simulink library "MX_Library"  (Simulink 7.7)
settings: Solver=ode45  StartTime=0.0  StopTime=10.0  RelTol=1e-3
values from neighbouring files (symbols this model uses):
  ACTIVE = Bobcat.Parameter; CreateDefine( ACTIVE                         ,1                          ,'Define' ,'defines.h' )    [defines.m]
  CD_PRECISION_REF_NOMINAL_VALUE = Bobcat.Parameter; CreateAliasCD( CD_PRECISION_REF_NOMINAL_VALUE                       ,uint16(511)                ,'ConstantDataPointer' ,'CONSTANT_DATA' ,'PRECISION_REF_NOMINAL_VALUE')    [cdata.m]
  ENGINE_CRANKING = Bobcat.Parameter; CreateDefine( ENGINE_CRANKING                ,2                          ,'Define' ,'defines.h' )    [defines.m]
  ERROR_OFF = Bobcat.Parameter; CreateDefine( ERROR_OFF                      ,3                          ,'Define' ,'defines.h' )    [defines.m]
  ERROR_ON = Bobcat.Parameter; CreateDefine( ERROR_ON                       ,2                          ,'Define' ,'defines.h' )    [defines.m]
  FAILURE = Bobcat.Parameter; CreateDefine( FAILURE                        ,28                         ,'Define' ,'defines.h' )    [defines.m]
  FULL_ON = Bobcat.Parameter; CreateDefine( FULL_ON                        ,fi(0,0,16,16,'hex','ffff') ,'Define' ,'defines.h' )    [defines.m]
  INACTIVE = Bobcat.Parameter; CreateDefine( INACTIVE                       ,0                          ,'Define' ,'defines.h' )    [defines.m]
  NON_FUNCTIONAL = Bobcat.Parameter; CreateDefine( NON_FUNCTIONAL                 ,255                        ,'Define' ,'defines.h' )    [defines.m]
  NORMAL = Bobcat.Parameter; CreateDefine( NORMAL                         ,8                          ,'Define' ,'defines.h' )    [defines.m]
  OORL = Bobcat.Parameter; CreateDefine( OORL                           ,22                         ,'Define' ,'defines.h' )    [defines.m]
  OPEN_CIRCUIT = Bobcat.Parameter; CreateDefine( OPEN_CIRCUIT                   ,7                          ,'Define' ,'defines.h' )    [defines.m]
  OPEN_STG = Bobcat.Parameter; CreateDefine( OPEN_STG                       ,31                         ,'Define' ,'defines.h' )    [defines.m]
  OVERCURRENT = Bobcat.Parameter; CreateDefine( OVERCURRENT                    ,32                         ,'Define' ,'defines.h' )    [defines.m]
  RESET = Bobcat.Parameter; CreateDefine( RESET                          ,2                          ,'Define' ,'defines.h' )    [defines.m]
  SHORT_TO_BATTERY = Bobcat.Parameter; CreateDefine( SHORT_TO_BATTERY               ,5                          ,'Define' ,'defines.h' )    [defines.m]
  SHORT_TO_GROUND = Bobcat.Parameter; CreateDefine( SHORT_TO_GROUND                ,6                          ,'Define' ,'defines.h' )    [defines.m]
  srate = 0.010    (= 0.01)    [LoadWorkspace.m]
  UNLIMITED = Bobcat.Parameter; CreateDefine( UNLIMITED                      ,65535                      ,'Define' ,'defines.h' )    [defines.m]
undefined symbols (not defined in the file or in its folder): BIDIRECTIONAL_CTRL, CD__AFBK_GAIN, CD__DEBOUNCE_OPEN_CIRCUIT, CD__DEBOUNCE_OVERCURRENT, CD__DEBOUNCE_SHORT_TO_BATTERY, CD__DEBOUNCE_SHORT_TO_GROUND, CD__ENABLE_AFBK_GAIN, CD__ENABLE_DEBOUNCE_OPEN_CIRCUIT, CD__ENABLE_DEBOUNCE_OVERCURRENT, CD__ENABLE_DEBOUNCE_SHORT_TO_BATTERY, CD__ENABLE_DEBOUNCE_SHORT_TO_GROUND, CD__ENABLE_FEEDBACK_FUNCTION, CD__ENABLE_IFBK_GAIN, CD__ENABLE_MAX_VOLTS, CD__ENABLE_NON_ZERO_CURRENT, CD__ENABLE_NON_ZERO_DUTY, CD__ENABLE_OVERCURRENT, CD__FUNCTION, CD__IFBK_GAIN, CD__KI, CD__KP, CD__MAX_VOLTS, CD__NON_ZERO_CURRENT, CD__NON_ZERO_DUTY, CD__OVERCURRENT, DEBOUNCE_ERROR_OFF, DEBOUNCE_ERROR_ON, DiscIntNeverNeededParam, FN_, IFBK_MAX, KI, KP, MAX_VOLTS, NZ_DUTY, NZ_IFBK, OC_DB_CNT, OPEN_DB_CNT, OSTG_DB_CNT, STB_DB_CNT, STG_DB_CNT
libraries: simulink x12, MX_Library x11
(part 1 of 2)
settings Model: Creator=alliebel  LastModifiedBy=aliebel

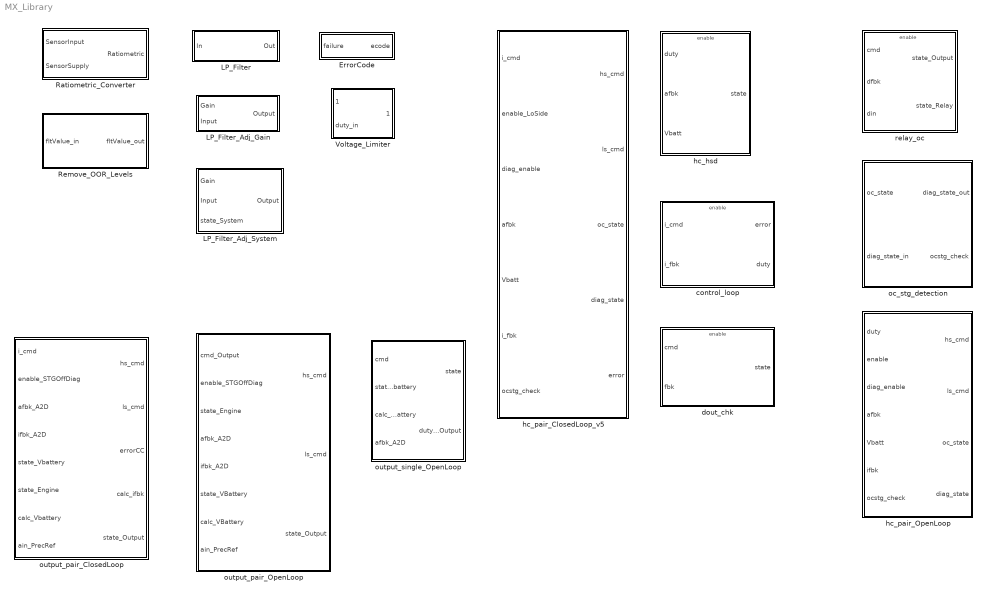
== system MX_Library ==
  ErrorCode : Subsystem  TreatAsAtomicUnit=on  RTWFileName=mod_Library  mask{FUNCTION=FN_}
      settings: AttributesFormatString=FUNCTION=%<FUNCTION>  RTWFcnNameOpts=Use subsystem name  RTWFileNameOpts=User specified
  LP_Filter : Subsystem  TreatAsAtomicUnit=on  RTWFcnName=LP_Filter  RTWFileName=mod_Library  mask{GAIN=3}
      mask prompts: GAIN "Gain for filter"
      settings: RTWFcnNameOpts=Use subsystem name  RTWFileNameOpts=User specified
  LP_Filter_Adj_Gain : Subsystem  TreatAsAtomicUnit=on  RTWFileName=mod_Library
      settings: RTWFcnNameOpts=Use subsystem name  RTWFileNameOpts=User specified
  LP_Filter_Adj_System : Subsystem  TreatAsAtomicUnit=on  RTWFileName=mod_Library
      settings: RTWFcnNameOpts=Use subsystem name  RTWFileNameOpts=User specified
  Ratiometric_Converter : Subsystem  TreatAsAtomicUnit=on  RTWFileName=mod_Library  mask{multiplier=1000}
      mask prompts: multiplier "Ratiometric Multiplier"
      settings: RTWFcnNameOpts=Use subsystem name  RTWFileNameOpts=User specified
  Remove_OOR_Levels : Subsystem  TreatAsAtomicUnit=on  RTWFileName=mod_Library  mask{OORL_LEVEL=50, OORH_LEVEL=950}
      settings: RTWFcnNameOpts=Use subsystem name  RTWFileNameOpts=User specified
  Voltage_Limiter : Subsystem  TreatAsAtomicUnit=on  RTWFileName=mod_Library
      settings: RTWFileNameOpts=User specified
  control_loop : Subsystem  TreatAsAtomicUnit=on  RTWFileName=mod_Library  mask{KP=KP, KI=KI}
      mask prompts: KP "Proportional Gain (Kp) -storage: fi(1,16,15)"; KI "Integral Gain (Ki) -storage: fi(1,16,15)"
      settings: RTWFcnNameOpts=Use subsystem name  RTWFileNameOpts=User specified
  dout_chk : Subsystem  TreatAsAtomicUnit=on  mask(Low Current, Low Side Driver -Monitor){ERR_ON_DB_CNT=DEBOUNCE_ERROR_ON, ERR_OFF_DB_CNT=DEBOUNCE_ERROR_OFF}
      mask prompts: ERR_ON_DB_CNT "Error On debounce count (10mS/count)"; ERR_OFF_DB_CNT "Error Off debounce count (10mS/count)"
      mask help:
      | Inputs:
      |   cmd: current output command (0-off, 1-on)
      |       storage: boolean
      |
      |   fbk: current output feedback (0-off, 1-on)
      |       storage: boolean
      |
      | Outputs:
      |   state:   8-bit value representing driver state
      |             (8) -> OK
      |             (2) -> error on   // cmd==off, fbk==on
      |             (3) -> error off  // cmd==on,  fbk==off
      mask Help: This block monitors the state of a digital output.
  hc_hsd : Subsystem  TreatAsAtomicUnit=on  RTWFileName=mod_Library  mask(High Current, High Side Driver -Monitor){STB_DB_CNT=STB_DB_CNT, STG_DB_CNT=STG_DB_CNT, OPEN_DB_CNT=OPEN_DB_CNT}
      mask prompts: STB_DB_CNT "Short to Battery (STB) debounce count"; STG_DB_CNT "Short to Ground (STG) debounce count"; OPEN_DB_CNT "Open circuit debounce count"
      mask help:
      | Inputs:
      |     duty: current output command (pwm %,  0-off, 1-on)
      |            storage:  ufix(16) - 100 / (2^16-1) percent per bit.
      |
      |     afbk:  high side analog feedback (volts)
      |            storage:  ufix(16) - 1 / (2^8)  volts per bit.
      |
      |     Vbatt: battery potential (volts)
      |            storage:  ufix(16) - 1 / (2^8)  volts per bit.
      |
      | Outputs:
      |     state:  8-bit value representing detected fault condition.
      |                (8) -> OK, output operating properly.
      |                (5) -> STB, short to battery
      |                (6) -> STG, short to ground
      |                (7) -> OPEN, open circuit
      settings: RTWFcnNameOpts=Use subsystem name  RTWFileNameOpts=User specified
      mask Help:
      | This block monitors the feedbacks associated with a "hc_hsd" (hig-current high-side-driver) and reports any faults associated with the output.
      | 
      | Parameter storage.
      | 
      | STB_DB_CNT : ufix(16) - 0.01 seconds per bit.
  hc_pair_ClosedLoop_v5 : Subsystem  TreatAsAtomicUnit=on  RTWFileName=mod_Library  mask{IFBK_MAX=IFBK_MAX, NZ_IFBK=NZ_IFBK, NZ_DUTY=NZ_DUTY, STB_DB_CNT=STB_DB_CNT, OPEN_DB_CNT=OPEN_DB_CNT, OSTG_DB_CNT=OSTG_DB_CNT, STG_DB_CNT=STG_DB_CNT, OC_DB_CNT=OC_DB_CNT, KP=KP, KI=KI, BIDIRECTIONAL_CTRL=BIDIRECTIONAL_CTRL}
      mask prompts: IFBK_MAX "Over Current Limit (Amps)  -storage uint(16), 1/2^12 amps per bit."; NZ_IFBK "Non-Zero Current (Amps) -storage uint(16), 1/2^12 amps per bit"; NZ_DUTY "Non-Zero Duty Cycle (%) -storage uint(16) 100/2^16 % per bit"; STB_DB_CNT "Short To Battery (STB) debounce count -storage uint(16)"; OPEN_DB_CNT "Open debounce count (10mS/count) -storage uint(16)"; OSTG_DB_CNT "Open or Short to Ground (OSTG) debounce count  -storage uint(16)"; STG_DB_CNT "Short To Ground (STG) debounce count -storage uint(16)"; OC_DB_CNT "Over Current (OC) debounce count -storage uint(16)"; KP "Kp  -storage: fi(1,16,15)"; KI "Ki    -storage: fi(1,16,15)C"; BIDIRECTIONAL_CTRL "Bi-directional Current Control"
      mask help:
      | This block implements an open loop High/Low output pair.
      |
      | Inputs:
      |   i_cmd:   command (Amps)...   storage:  ufix(16) - 1/ (2^12) Amps per bit.
      |   enable:    state of output (0-off, 1-on)...   storage: boolean.
      |   diag_enable:    state of diagnostics (0-off, 1-on)...   storage: boolean
      |   afbk:    high side analog feedback (volts)... storage: uint(16) 1/2^8 volts per bit
      |   Vbatt:   battery potential (volts)... storage: uint(16) 1/2^8 volts per bit
      |   ifbk:    low side current feedback (amps)... storage: uint(16) 1/2^12 amps per bit
      |
      | Outputs:
      |     hs_cmd: (pwm%, 0-off, 1-on)...   storage:  ufix(16) - 100/ (2^16-1) percent per bit.
      |     ls_cmd:  (boolean)... storage: boolean
      |     oc_state: state of the over-current detection mechanism.
      |                 (8)  -> Ok
      |                 (32) -> error, too much current sensed flowing through this output
      |                                      output is turned off...
      |
      |   diag_state:  state of the general fault state monitoring.
      |                 (8)  -> Ok
      |                 (5)  -> STB, Short to battery
      |                 (6)  -> STG, Short to ground
      |                 (7)  -> Open, open circuit
      |                 (31) -> OSTG, open or short to ground
      settings: RTWFcnNameOpts=Use subsystem name  RTWFileNameOpts=User specified
  hc_pair_OpenLoop : Subsystem  TreatAsAtomicUnit=on  RTWFileName=mod_Library  mask(hc_pair output){IFBK_MAX=IFBK_MAX, NZ_IFBK=NZ_IFBK, NZ_DUTY=NZ_DUTY, STB_DB_CNT=STB_DB_CNT, OPEN_DB_CNT=OPEN_DB_CNT, OSTG_DB_CNT=OSTG_DB_CNT, STG_DB_CNT=STG_DB_CNT, OC_DB_CNT=OC_DB_CNT}
      mask prompts: IFBK_MAX "Over-Current shutdown limit (Amps)  -storage: uint(16) 1/2^12 amps/bit"; NZ_IFBK "Non-Zero current feedback (Amps) -storage: uint(16) 1/2^12 amps/bit"; NZ_DUTY "Non-Zero duty cycle (% duty) -storage uint(16) 100/2^16 % per bit."; STB_DB_CNT "Short to Battey (STB) debounce count -storage uint(16)"; OPEN_DB_CNT "Open debounce count -storage uint(16)"; OSTG_DB_CNT "Open or short to Ground (OSTG) debounce count -storage uint(16)"; STG_DB_CNT "Short to Ground (STG) debounce count -storage uint(16)"; OC_DB_CNT "Overcurrent debounce count -storage uint(16)"
      mask help:
      | This block implements an open loop High/Low output pair.
      |
      | Inputs:
      |   duty:    pwm%, 0-off, 1-on)...   storage:  ufix(16) - 100/ (2^16-1) percent per bit.
      |   enable:    state of output (0-off, 1-on)...   storage: boolean.
      |   diag_enable:    state of diagnostics (0-off, 1-on)...   storage: boolean
      |   afbk:    high side analog feedback (volts)... storage: uint(16) 1/2^8 volts per bit
      |   Vbatt:   battery potential (volts)... storage: uint(16) 1/2^8 volts per bit
      |   ifbk:    low side current feedback (amps)... storage: uint(16) 1/2^12 amps per bit
      |
      | Outputs:
      |     hs_cmd: (pwm%, 0-off, 1-on)...   storage:  ufix(16) - 100/ (2^16-1) percent per bit.
      |     ls_cmd:  (boolean)... storage: boolean
      |     oc_state: state of the over-current detection mechanism.
      |                 (8)  -> Ok
      |                 (32) -> error, too much current sensed flowing through this output
      |                                      output is turned off...
      |
      |   diag_state:  state of the general fault state monitoring.
      |                 (8)  -> Ok
      |                 (5)  -> STB, Short to battery
      |                 (6)  -> STG, Short to ground
      |                 (7)  -> Open, open circuit
      |                 (31) -> OSTG, open or short to ground
      settings: RTWFcnNameOpts=Use subsystem name  RTWFileNameOpts=User specified
  oc_stg_detection : Subsystem  TreatAsAtomicUnit=on  RTWFileName=mod_Library  mask{CD_DEBOUNCE_OPEN_CIRCUIT=OPEN_DB_CNT, CD_DEBOUNCE_SHORT_TO_GROUND=STG_DB_CNT}
      mask prompts: CD_DEBOUNCE_OPEN_CIRCUIT "Debounce Open Circuit"; CD_DEBOUNCE_SHORT_TO_GROUND "Debounce Short to Ground"
      settings: RTWFcnNameOpts=Use subsystem name  RTWFileNameOpts=User specified
  output_pair_ClosedLoop : Subsystem  TreatAsAtomicUnit=on  RTWFileName=mod_Library  mask{AFBK_GAIN=CD__AFBK_GAIN, IFBK_GAIN=CD__IFBK_GAIN, OPEN_DB_CNT=CD__DEBOUNCE_OPEN_CIRCUIT, STG_DB_CNT=CD__DEBOUNCE_SHORT_TO_GROUND, OSTG_DB_CNT=CD__DEBOUNCE_SHORT_TO_GROUND, STB_DB_CNT=CD__DEBOUNCE_SHORT_TO_BATTERY, OC_DB_CNT=CD__DEBOUNCE_OVERCURRENT, IFBK_MAX=CD__OVERCURRENT, NZ_IFBK=CD__NON_ZERO_CURRENT, NZ_DUTY=CD__NON_ZERO_DUTY, KP=CD__KP, KI=CD__KI, BIDIRECTIONAL_CTRL=NON_FUNCTIONAL}
      mask prompts: AFBK_GAIN "Analog Feedback Gain -storage: fi(0,16,8)"; IFBK_GAIN "Current Feedback Gain  -storage: fi(0,16,16)"; OPEN_DB_CNT "Debounce Open Circuit  -storage: uint(16)"; STG_DB_CNT "Debounce STG  -storage uint(16)"; OSTG_DB_CNT "Debounce Open or STG -storage uint(16)"; STB_DB_CNT "Debounce STB -storage uint(16)"; OC_DB_CNT "Debounce Overcurrent -storage uint(16)"; IFBK_MAX "Overcurrent Shutdown limit -storage: fi(0,16,12)"; NZ_IFBK "Non-zero Current Feedback -storage: fi(0,16,12)"; NZ_DUTY "Non-zero Duty Cycle -storage: fi(0,16,16)"; KP "Proportional Gain (Kp) - storage: fi(1,16,15)"; KI "Integral Gain (Ki) - storage: fi(1,16,15)"; BIDIRECTIONAL_CTRL "Bi-Directional Current Control"
      settings: RTWFcnNameOpts=Use subsystem name  RTWFileNameOpts=User specified
  output_pair_OpenLoop : Subsystem  TreatAsAtomicUnit=on  RTWFileName=mod_Library  mask{FEEDBACK_ENABLE=CD__ENABLE_FEEDBACK_FUNCTION, AFBK_GAIN=CD__ENABLE_AFBK_GAIN, IFBK_GAIN=CD__ENABLE_IFBK_GAIN, OPEN_DB_CNT=CD__ENABLE_DEBOUNCE_OPEN_CIRCUIT, STG_DB_CNT=CD__ENABLE_DEBOUNCE_SHORT_TO_GROUND, STB_DB_CNT=CD__ENABLE_DEBOUNCE_SHORT_TO_BATTERY, OC_DB_CNT=CD__ENABLE_DEBOUNCE_OVERCURRENT, OSTG_DB_CNT=CD__ENABLE_DEBOUNCE_SHORT_TO_GROUND, IFBK_MAX=CD__ENABLE_OVERCURRENT, NZ_IFBK=CD__ENABLE_NON_ZERO_CURRENT, NZ_DUTY=CD__ENABLE_NON_ZERO_DUTY, MAX_VOLTS=CD__ENABLE_MAX_VOLTS}
      mask prompts: FEEDBACK_ENABLE "Feedback Enable:"; AFBK_GAIN "Analog Feedback Gain -storage: fi(0,16,8)"; IFBK_GAIN "Current Feedback Gain  -storage: fi(0,16,16)"; OPEN_DB_CNT "Debounce Open Circuit  -storage: uint(16)"; STG_DB_CNT "Debounce STG  -storage uint(16)"; STB_DB_CNT "Debounce STB -storage uint(16)"; OC_DB_CNT "Debounce Overcurrent -storage uint(16)"; OSTG_DB_CNT "Debounce Open or STG -storage uint(16)"; IFBK_MAX "Overcurrent Shutdown limit -storage: fi(0,16,12)"; NZ_IFBK "Non-zero Current Feedback -storage: fi(0,16,12)"; NZ_DUTY "Non-zero Duty Cycle -storage: fi(0,16,16)"; MAX_VOLTS "Maximum Voltage Limit"
      settings: RTWFcnNameOpts=Use subsystem name  RTWFileNameOpts=User specified
  output_single_OpenLoop : Subsystem  TreatAsAtomicUnit=on  RTWFileName=mod_Library  mask{FUNCTION=CD__FUNCTION, AFBK_GAIN=CD__AFBK_GAIN, OPEN_DB_CNT=CD__DEBOUNCE_OPEN_CIRCUIT, STB_DB_CNT=CD__DEBOUNCE_SHORT_TO_BATTERY, STG_DB_CNT=CD__DEBOUNCE_SHORT_TO_GROUND, MAX_VOLTS=CD__MAX_VOLTS}
      mask prompts: FUNCTION "Functional:"; AFBK_GAIN "Analog Feedback Gain: -storage: fi(0,16,8)"; OPEN_DB_CNT "Debounce Open Circuit: -storage: uint(16)"; STB_DB_CNT "Debounce STB: -storage: uint(16)"; STG_DB_CNT "Debounce STG: -storage: uint(16)"; MAX_VOLTS "Maximum Voltage Limit"
      settings: RTWFcnNameOpts=Use subsystem name  RTWFileNameOpts=User specified
  relay_oc : Subsystem  TreatAsAtomicUnit=on  RTWFileName=mod_Library  mask(relay moniitor){ERROR_ON_DB_CNT=40, ERROR_OFF_DB_CNT=40, NORMAL_DB_CNT=40}
      mask prompts: ERROR_ON_DB_CNT "dfbk Error on debounce count"; ERROR_OFF_DB_CNT "dfbk Error off debounce count"; NORMAL_DB_CNT "dfbk normal debounce count"
      mask help:
      | Often "lc_lsd" outputs are used to drive relays.  If this is the case the output of the relay is fed back to a digital input (din) to monitor the relay function.  This block adds the relay output monitor to the "lc_lsd" monitor to create a "relay" monitor.
      |
      | Inputs:
      |   cmd: output command (0-off, 1-on)
      |       storage: boolean
      |
      |   dfbk: output feedback (0-off, 1-on)
      |       storage: boolean
      |
      |   din: relay output feedback (0-off, 1-on)
      |       storage: boolean
      |
      | Outputs:
      |   state:   8-bit value representing driver state
      |             (8) -> OK
      |             (2) -> error on   // cmd==off, dfbk==on
      |             (3) -> error off  // cmd==on,  dfbk==off
      |
      |   din_state:   8-bit value representing driver state
      |             (8) -> OK
      |             (2) -> error on   // cmd==off, din==on
      |             (3) -> error off  // cmd==on,  din==off
      settings: RTWFcnNameOpts=Use subsystem name  RTWFileNameOpts=User specified

== system MX_Library/ErrorCode ==
  failure : Inport  OutDataTypeStr=uint8
  Constant : Constant  Value=256  OutDataTypeStr=uint16
  Constant1 : Constant  Value=FUNCTION  OutDataTypeStr=uint16
  Product : Product  OutDataTypeStr=uint16  RndMeth=Zero
  Sum : Sum  OutDataTypeStr=uint16
  ecode : Outport  OutDataTypeStr=uint16
  wires:
  Constant/1 -> Product/2
  Constant1/1 -> Product/1
  Product/1 -> Sum/2
  failure/1 -> Sum/1
  Sum/1 -> ecode/1

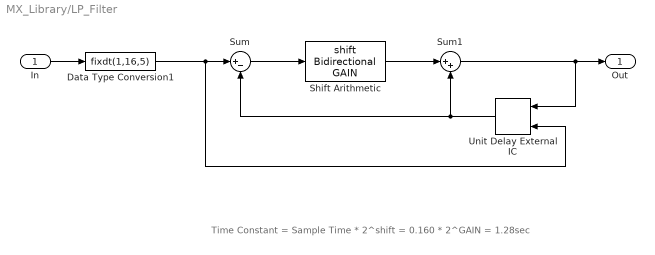
== system MX_Library/LP_Filter ==
  note: Time Constant = Sample Time * 2^shift
      | = 0.160 * 2^GAIN = 1.28sec
  In : Inport
  Data Type Conversion1 : DataTypeConversion  OutMin=0  OutMax=1023  OutDataTypeStr=fixdt(1,16,5)
  Shift Arithmetic : ArithShift  BitShiftNumber=GAIN
  Sum : Sum  Inputs=|+-  OutDataTypeStr=fixdt(1,16,5)  SaturateOnIntegerOverflow=on
  Sum1 : Sum  Inputs=|++  OutDataTypeStr=fixdt(1,16,5)  SaturateOnIntegerOverflow=on
  Unit Delay External IC : simulink/Additional Math & Discrete/Additional Discrete/Unit Delay External IC  SystemSampleTime=-1  tsamp=-1
  Out : Outport
  wires:
  Sum/1 -> Shift Arithmetic/1
  Sum1/1 -> Unit Delay External IC/1, Out/1
  Shift Arithmetic/1 -> Sum1/1
  Unit Delay External IC/1 -> Sum1/2, Sum/2
  In/1 -> Data Type Conversion1/1
  Data Type Conversion1/1 -> Sum/1, Unit Delay External IC/2

== system MX_Library/LP_Filter_Adj_Gain ==
  Gain : Inport
  Input : Inport  Port=2
  LP_Filter_Adj_Gain : Stateflow chart  RTWFileName=mod_Library
  Output : Outport
  wires:
  LP_Filter_Adj_Gain/1(Output) -> Output/1
  Input/1 -> LP_Filter_Adj_Gain/2(Input)
  Gain/1 -> LP_Filter_Adj_Gain/1(Gain)

== system MX_Library/LP_Filter_Adj_System ==
  Gain : Inport
  Input : Inport  Port=2
  state_System : Inport  Port=3
  LP_Fitler_Adj_Gain : Stateflow chart  TreatAsAtomicUnit=on
  Output : Outport
  wires:
  state_System/1 -> LP_Fitler_Adj_Gain/3(state_System)
  Gain/1 -> LP_Fitler_Adj_Gain/1(Gain)
  Input/1 -> LP_Fitler_Adj_Gain/2(Input)
  LP_Fitler_Adj_Gain/1(Output) -> Output/1

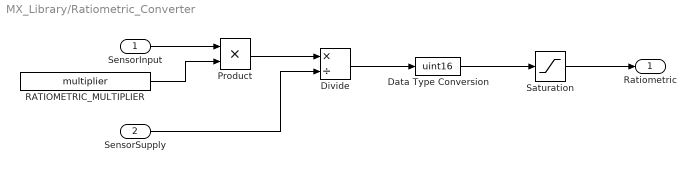
== system MX_Library/Ratiometric_Converter ==
  SensorInput : Inport
  SensorSupply : Inport  Port=2
  Data Type Conversion : DataTypeConversion  OutDataTypeStr=uint16
  Divide : Product  Inputs=*/  OutDataTypeStr=uint32
  Product : Product  OutDataTypeStr=uint32  InputSameDT=on
  RATIOMETRIC_MULTIPLIER : Constant  Value=multiplier  OutDataTypeStr=uint16
  Saturation : Saturate  UpperLimit=2047  LowerLimit=0
  Ratiometric : Outport
  wires:
  Divide/1 -> Data Type Conversion/1
  SensorSupply/1 -> Divide/2
  Product/1 -> Divide/1
  RATIOMETRIC_MULTIPLIER/1 -> Product/2
  SensorInput/1 -> Product/1
  Data Type Conversion/1 -> Saturation/1
  Saturation/1 -> Ratiometric/1

== system MX_Library/Remove_OOR_Levels ==
  fltValue_in : Inport
  RemoveOORLevels : Stateflow chart  TreatAsAtomicUnit=on
  fltValue_out : Outport
  wires:
  RemoveOORLevels/1(fltValue_out) -> fltValue_out/1
  fltValue_in/1 -> RemoveOORLevels/1(fltValue_in)

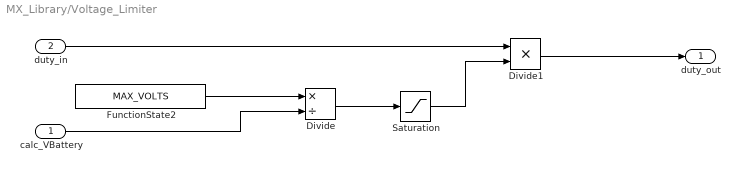
== system MX_Library/Voltage_Limiter ==
  calc_VBattery : Inport
  duty_in : Inport  Port=2
  Divide : Product  Inputs=*/  OutDataTypeStr=fixdt(0,16,12)  RndMeth=Simplest  SaturateOnIntegerOverflow=on  LockScale=on
  Divide1 : Product  Inputs=**  OutDataTypeStr=fixdt(0,16,16)  RndMeth=Simplest  SaturateOnIntegerOverflow=on  LockScale=on
  FunctionState2 : Constant  Value=MAX_VOLTS  OutDataTypeStr=fixdt(0,16,8)
  Saturation : Saturate  UpperLimit=1  LowerLimit=0
  duty_out : Outport
  wires:
  Divide1/1 -> duty_out/1
  duty_in/1 -> Divide1/1
  calc_VBattery/1 -> Divide/2
  Saturation/1 -> Divide1/2
  Divide/1 -> Saturation/1
  FunctionState2/1 -> Divide/1

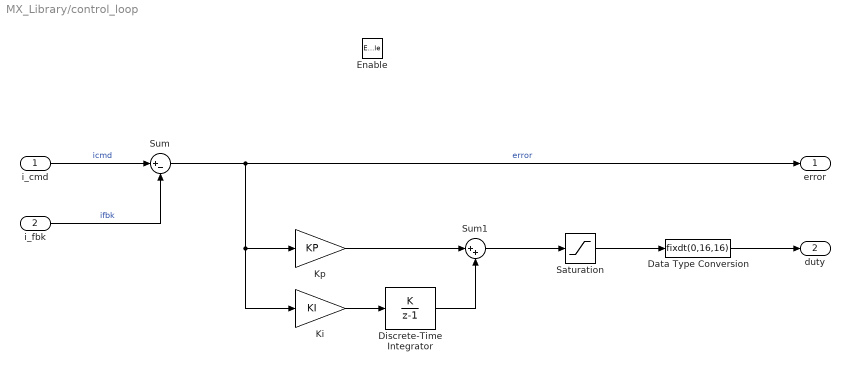
== system MX_Library/control_loop ==
  i_cmd : Inport
  i_fbk : Inport  Port=2
  Enable : EnablePort  StatesWhenEnabling=reset
  Data Type Conversion : DataTypeConversion  OutDataTypeStr=fixdt(0,16,16)  RndMeth=Nearest  SaturateOnIntegerOverflow=on  LockScale=on
  Discrete-Time Integrator : DiscreteIntegrator  IntegratorMethod=Accumulation: Forward Euler  gainval=1  InitialConditionMode=State only (most efficient)  SampleTime=-1  LimitOutput=on  UpperSaturationLimit=1  LowerSaturationLimit=-1  ICPrevOutput=DiscIntNeverNeededParam  ICPrevScaledInput=DiscIntNeverNeededParam
  Ki : Gain  Gain=KI  ParamDataTypeStr=fixdt(1,16,15)  OutDataTypeStr=fixdt(1,16,14)  RndMeth=Nearest  SaturateOnIntegerOverflow=on  LockScale=on
  Kp : Gain  Gain=KP  ParamDataTypeStr=fixdt(1,16,15)  OutDataTypeStr=fixdt(1,16,14)  RndMeth=Nearest  SaturateOnIntegerOverflow=on  LockScale=on
  Saturation : Saturate  UpperLimit=1  LowerLimit=0
  Sum : Sum  Inputs=|+-  AccumDataTypeStr=fixdt(1,16,11)  OutDataTypeStr=fixdt(1,16,11)  RndMeth=Nearest  SaturateOnIntegerOverflow=on  LockScale=on
  Sum1 : Sum  Inputs=|++
  error : Outport  OutputWhenDisabled=reset  InitialOutput=0
  duty : Outport  Port=2  OutputWhenDisabled=reset  InitialOutput=0
  wires:
  Ki/1 -> Discrete-Time Integrator/1
  i_fbk/1 -> Sum/2  "ifbk"
  Saturation/1 -> Data Type Conversion/1
  i_cmd/1 -> Sum/1  "icmd"
  Data Type Conversion/1 -> duty/1
  Sum/1 -> error/1, Kp/1, Ki/1  "error"
  Sum1/1 -> Saturation/1
  Kp/1 -> Sum1/1
  Discrete-Time Integrator/1 -> Sum1/2

== system MX_Library/dout_chk ==
  note: Inputs:
      |     cmd:  desired output (boolean)
      |
      |     fbk:  digital feedback on output pin (boolean)
      |
      | Outputs:
      |     state:   8-bit value representing driver state
      |             (8) -> ok
      |             (2) -> error on   // cmd==off, fbk==on
      |             (3) -> error off  // cmd==on,  fbk==off
  cmd : Inport  OutDataTypeStr=boolean
  fbk : Inport  Port=2  OutDataTypeStr=boolean
  Enable : EnablePort  StatesWhenEnabling=reset
  Fault monitor : Stateflow chart  TreatAsAtomicUnit=on
  state : Outport  OutDataTypeStr=uint8  OutputWhenDisabled=reset  InitialOutput=[8]
  wires:
  cmd/1 -> Fault monitor/1(cmd)
  fbk/1 -> Fault monitor/2(fbk)
  Fault monitor/1(state) -> state/1

== system MX_Library/hc_hsd ==
  duty : Inport  OutDataTypeStr=fixdt(0,16,16)
  afbk : Inport  Port=2  OutDataTypeStr=fixdt(0,16,8)
  Vbatt : Inport  Port=3  OutDataTypeStr=fixdt(0,16,8)
  Enable : EnablePort  StatesWhenEnabling=reset
  Divide : Product  Inputs=*/  OutDataTypeStr=fixdt(1,16,8)  RndMeth=Simplest  LockScale=on
  Fault monitor : Stateflow chart
  state : Outport  OutDataTypeStr=uint8  OutputWhenDisabled=reset  InitialOutput=[8]
  wires:
  duty/1 -> Fault monitor/1(hs_cmd)  "duty"
  Divide/1 -> Fault monitor/2(afbk_ratio)  "afbk_ratio"
  Vbatt/1 -> Divide/2  "Vbatt"
  afbk/1 -> Divide/1  "afbk"
  Fault monitor/1(state) -> state/1  "state"

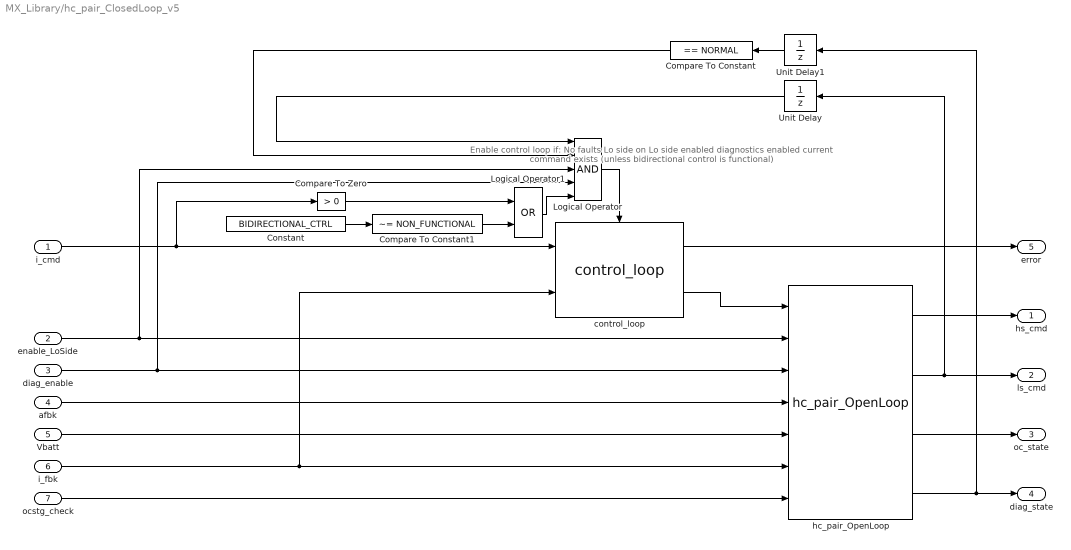
== system MX_Library/hc_pair_ClosedLoop_v5 ==
  note: Enable control loop if:
      | No faults
      | Lo side on
      | Lo side enabled
      | diagnostics enabled
      | current command exists (unless bidirectional control is functional)
  i_cmd : Inport  OutDataTypeStr=fixdt(0,16,12)
  enable_LoSide : Inport  Port=2  OutDataTypeStr=boolean
  diag_enable : Inport  Port=3  OutDataTypeStr=boolean
  afbk : Inport  Port=4  OutDataTypeStr=fixdt(0,16,8)
  Vbatt : Inport  Port=5  OutDataTypeStr=fixdt(0,16,8)
  i_fbk : Inport  Port=6  OutDataTypeStr=fixdt(0,16,12)
  ocstg_check : Inport  Port=7
  Compare To Constant : simulink/Logic and Bit Operations/Compare To Constant  SystemSampleTime=-1  relop===  const=NORMAL  LogicOutDataTypeMode=boolean  ZeroCross=off
  Compare To Constant1 : simulink/Logic and Bit Operations/Compare To Constant  SystemSampleTime=-1  relop=~=  const=NON_FUNCTIONAL  LogicOutDataTypeMode=boolean
  Compare To Zero : simulink/Logic and Bit Operations/Compare To Zero  SystemSampleTime=-1  relop=>  LogicOutDataTypeMode=boolean
  Constant : Constant  Value=BIDIRECTIONAL_CTRL  OutDataTypeStr=uint8
  Logical Operator : Logic  Inputs=5  AllPortsSameDT=off  OutDataTypeStr=boolean
  Logical Operator1 : Logic  Operator=OR  AllPortsSameDT=off  OutDataTypeStr=boolean
  Unit Delay : UnitDelay  SampleTime=-1
  Unit Delay1 : UnitDelay  SampleTime=-1
  control_loop : MX_Library/control_loop  SystemSampleTime=-1  KP=KP  KI=KI
  hc_pair_OpenLoop : MX_Library/hc_pair_OpenLoop  SystemSampleTime=-1  IFBK_MAX=IFBK_MAX  NZ_IFBK=NZ_IFBK  NZ_DUTY=NZ_DUTY  STB_DB_CNT=STB_DB_CNT  OPEN_DB_CNT=OPEN_DB_CNT  OSTG_DB_CNT=OSTG_DB_CNT  STG_DB_CNT=STG_DB_CNT  OC_DB_CNT=OC_DB_CNT
  hs_cmd : Outport  OutDataTypeStr=fixdt(0,16,16)
  ls_cmd : Outport  Port=2  OutDataTypeStr=boolean
  oc_state : Outport  Port=3  OutDataTypeStr=uint8
  diag_state : Outport  Port=4  OutDataTypeStr=uint8
  error : Outport  Port=5
  wires:
  ocstg_check/1 -> hc_pair_OpenLoop/7
  hc_pair_OpenLoop/1 -> hs_cmd/1
  hc_pair_OpenLoop/2 -> ls_cmd/1, Unit Delay/1
  hc_pair_OpenLoop/3 -> oc_state/1
  hc_pair_OpenLoop/4 -> Unit Delay1/1, diag_state/1
  i_cmd/1 -> control_loop/1, Compare To Zero/1
  i_fbk/1 -> hc_pair_OpenLoop/6, control_loop/2
  diag_enable/1 -> hc_pair_OpenLoop/3, Logical Operator/4
  afbk/1 -> hc_pair_OpenLoop/4
  Vbatt/1 -> hc_pair_OpenLoop/5
  Unit Delay/1 -> Logical Operator/1
  Unit Delay1/1 -> Compare To Constant/1
  Compare To Constant/1 -> Logical Operator/2
  Logical Operator/1 -> control_loop/Enable
  enable_LoSide/1 -> hc_pair_OpenLoop/2, Logical Operator/3
  control_loop/1 -> error/1
  control_loop/2 -> hc_pair_OpenLoop/1
  Compare To Zero/1 -> Logical Operator1/1
  Logical Operator1/1 -> Logical Operator/5
  Compare To Constant1/1 -> Logical Operator1/2
  Constant/1 -> Compare To Constant1/1

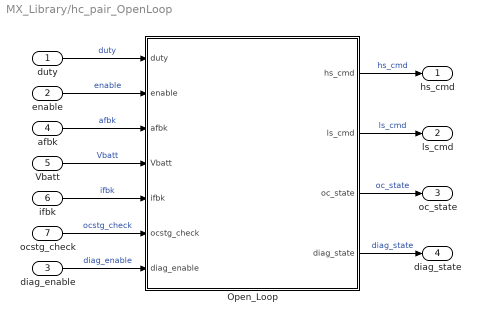
== system MX_Library/hc_pair_OpenLoop ==
  duty : Inport  OutDataTypeStr=fixdt(0,16,16)
  enable : Inport  Port=2  OutDataTypeStr=boolean
  diag_enable : Inport  Port=3  OutDataTypeStr=boolean
  afbk : Inport  Port=4  OutDataTypeStr=fixdt(0,16,8)
  Vbatt : Inport  Port=5  OutDataTypeStr=fixdt(0,16,8)
  ifbk : Inport  Port=6  OutDataTypeStr=fixdt(0,16,12)
  ocstg_check : Inport  Port=7
  Open_Loop : Subsystem
  hs_cmd : Outport  OutDataTypeStr=fixdt(0,16,16)
  ls_cmd : Outport  Port=2  OutDataTypeStr=boolean
  oc_state : Outport  Port=3  OutDataTypeStr=uint8
  diag_state : Outport  Port=4  OutDataTypeStr=uint8
  wires:
  diag_enable/1 -> Open_Loop/7(diag_enable)  "diag_enable"
  Open_Loop/4(diag_state) -> diag_state/1  "diag_state"
  Open_Loop/3(oc_state) -> oc_state/1  "oc_state"
  Open_Loop/2(ls_cmd) -> ls_cmd/1  "ls_cmd"
  Open_Loop/1(hs_cmd) -> hs_cmd/1  "hs_cmd"
  ocstg_check/1 -> Open_Loop/6(ocstg_check)  "ocstg_check"
  ifbk/1 -> Open_Loop/5(ifbk)  "ifbk"
  Vbatt/1 -> Open_Loop/4(Vbatt)  "Vbatt"
  afbk/1 -> Open_Loop/3(afbk)  "afbk"
  enable/1 -> Open_Loop/2(enable)  "enable"
  duty/1 -> Open_Loop/1(duty)  "duty"

== system MX_Library/oc_stg_detection ==
  oc_state : Inport
  diag_state_in : Inport  Port=2
  oc_operation_detection : Stateflow chart
  diag_state_out : Outport
  ocstg_check : Outport  Port=2
  wires:
  oc_operation_detection/2(ocstg_check) -> ocstg_check/1  "ocstg_check"
  oc_operation_detection/1(diag_state_out) -> diag_state_out/1  "diag_state_out"
  diag_state_in/1 -> oc_operation_detection/2(diag_state_in)  "diag_state_in"
  oc_state/1 -> oc_operation_detection/1(oc_state)  "oc_state"

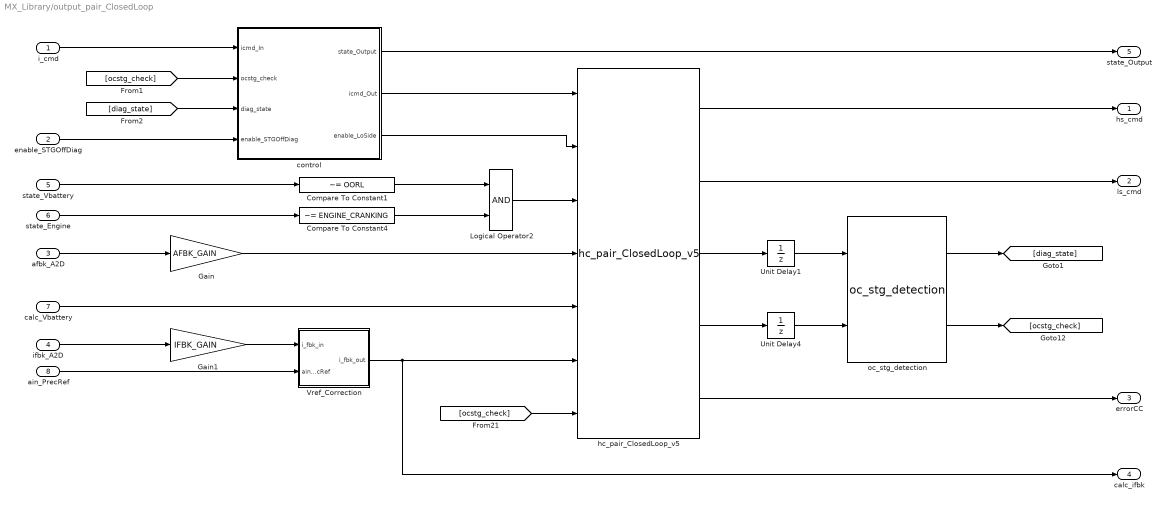
== system MX_Library/output_pair_ClosedLoop ==
  i_cmd : Inport
  enable_STGOffDiag : Inport  Port=2
  afbk_A2D : Inport  Port=3  OutDataTypeStr=uint16
  ifbk_A2D : Inport  Port=4  OutDataTypeStr=uint16
  state_Vbattery : Inport  Port=5
  state_Engine : Inport  Port=6
  calc_Vbattery : Inport  Port=7
  ain_PrecRef : Inport  Port=8  OutDataTypeStr=uint16
  Compare To Constant1 : simulink/Logic and Bit Operations/Compare To Constant  SystemSampleTime=-1  relop=~=  const=OORL  LogicOutDataTypeMode=boolean  ZeroCross=off
  Compare To Constant4 : simulink/Logic and Bit Operations/Compare To Constant  SystemSampleTime=-1  relop=~=  const=ENGINE_CRANKING  LogicOutDataTypeMode=boolean  ZeroCross=off
  Gain : Gain  Gain=AFBK_GAIN  ParamDataTypeStr=fixdt(0,16,8)  OutDataTypeStr=Inherit: Inherit via back propagation  SaturateOnIntegerOverflow=on
  Gain1 : Gain  Gain=IFBK_GAIN  ParamDataTypeStr=fixdt(0,16,16)  OutDataTypeStr=Inherit: Inherit via back propagation  SaturateOnIntegerOverflow=on
  Logical Operator2 : Logic  AllPortsSameDT=off  OutDataTypeStr=boolean
  Unit Delay1 : UnitDelay  SampleTime=-1
      settings: AttributesFormatString=<initial=%<X0>>\n<tsample=%<SampleTime>>
  Unit Delay4 : UnitDelay  SampleTime=-1
      settings: AttributesFormatString=<initial=%<X0>>\n<tsample=%<SampleTime>>
  Vref_Correction : Subsystem
  control : Stateflow chart  TreatAsAtomicUnit=on
  hc_pair_ClosedLoop_v5 : MX_Library/hc_pair_ClosedLoop_v5  SystemSampleTime=-1  IFBK_MAX=IFBK_MAX  NZ_IFBK=NZ_IFBK  NZ_DUTY=NZ_DUTY  STB_DB_CNT=STB_DB_CNT  OPEN_DB_CNT=OPEN_DB_CNT  OSTG_DB_CNT=OSTG_DB_CNT  STG_DB_CNT=STG_DB_CNT  OC_DB_CNT=OC_DB_CNT  KP=KP  KI=KI  BIDIRECTIONAL_CTRL=BIDIRECTIONAL_CTRL
  oc_stg_detection : MX_Library/oc_stg_detection  SystemSampleTime=-1  CD_DEBOUNCE_OPEN_CIRCUIT=OPEN_DB_CNT  CD_DEBOUNCE_SHORT_TO_GROUND=STG_DB_CNT
  hs_cmd : Outport
  ls_cmd : Outport  Port=2
  errorCC : Outport  Port=3
  calc_ifbk : Outport  Port=4
  state_Output : Outport  Port=5
  wires:
  hc_pair_ClosedLoop_v5/5 -> errorCC/1
  hc_pair_ClosedLoop_v5/2 -> ls_cmd/1
  Logical Operator2/1 -> hc_pair_ClosedLoop_v5/3
  Compare To Constant1/1 -> Logical Operator2/1
  state_Vbattery/1 -> Compare To Constant1/1
  Gain/1 -> hc_pair_ClosedLoop_v5/4
  afbk_A2D/1 -> Gain/1
  hc_pair_ClosedLoop_v5/1 -> hs_cmd/1
  state_Engine/1 -> Compare To Constant4/1
  Compare To Constant4/1 -> Logical Operator2/2
  Unit Delay4/1 -> oc_stg_detection/2
  Unit Delay1/1 -> oc_stg_detection/1
  hc_pair_ClosedLoop_v5/3 -> Unit Delay1/1
  hc_pair_ClosedLoop_v5/4 -> Unit Delay4/1
  calc_Vbattery/1 -> hc_pair_ClosedLoop_v5/5
  oc_stg_detection/2 -> [ocstg_check]
  [ocstg_check] -> hc_pair_ClosedLoop_v5/7
  i_cmd/1 -> control/1(icmd_In)
  control/2(icmd_Out) -> hc_pair_ClosedLoop_v5/1
  [ocstg_check] -> control/2(ocstg_check)
  control/3(enable_LoSide) -> hc_pair_ClosedLoop_v5/2
  control/1(state_Output) -> state_Output/1
  oc_stg_detection/1 -> [diag_state]
  [diag_state] -> control/3(diag_state)
  enable_STGOffDiag/1 -> control/4(enable_STGOffDiag)
  ain_PrecRef/1 -> Vref_Correction/2(ain_PrecRef)
  ifbk_A2D/1 -> Gain1/1
  Vref_Correction/1(i_fbk_out) -> calc_ifbk/1, hc_pair_ClosedLoop_v5/6
  Gain1/1 -> Vref_Correction/1(i_fbk_in)

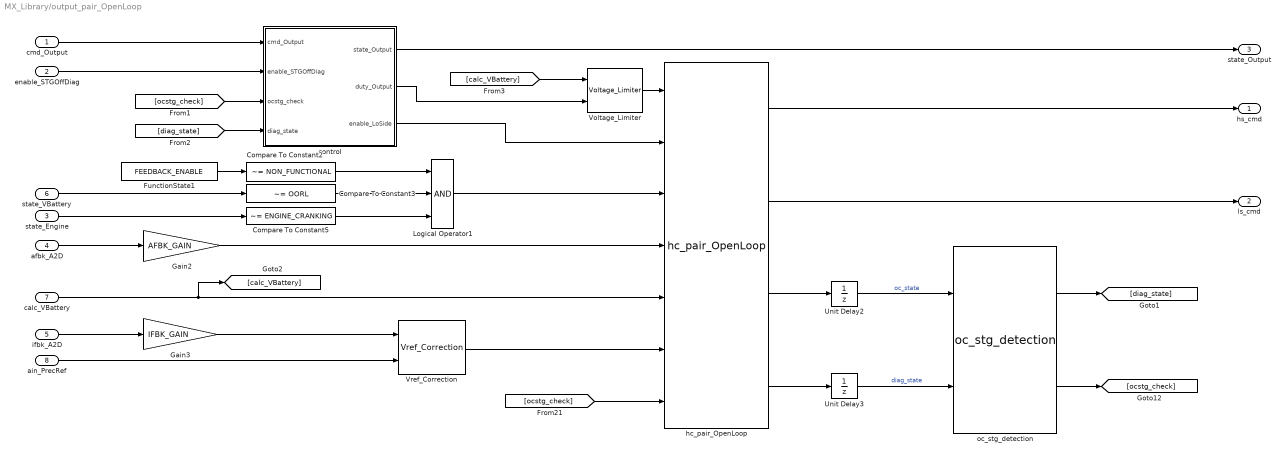
== system MX_Library/output_pair_OpenLoop ==
  cmd_Output : Inport
  enable_STGOffDiag : Inport  Port=2
  state_Engine : Inport  Port=3
  afbk_A2D : Inport  Port=4  OutDataTypeStr=uint16
  ifbk_A2D : Inport  Port=5  OutDataTypeStr=uint16
  state_VBattery : Inport  Port=6
  calc_VBattery : Inport  Port=7
  ain_PrecRef : Inport  Port=8  OutDataTypeStr=uint16
  Compare To Constant2 : simulink/Logic and Bit Operations/Compare To Constant  SystemSampleTime=-1  relop=~=  const=NON_FUNCTIONAL  LogicOutDataTypeMode=boolean  ZeroCross=off
  Compare To Constant3 : simulink/Logic and Bit Operations/Compare To Constant  SystemSampleTime=-1  relop=~=  const=OORL  LogicOutDataTypeMode=boolean  ZeroCross=off
  Compare To Constant5 : simulink/Logic and Bit Operations/Compare To Constant  SystemSampleTime=-1  relop=~=  const=ENGINE_CRANKING  LogicOutDataTypeMode=boolean  ZeroCross=off
  FunctionState1 : Constant  Value=FEEDBACK_ENABLE  OutDataTypeStr=uint8
  Gain2 : Gain  Gain=AFBK_GAIN  ParamDataTypeStr=fixdt(0,16,8)  OutDataTypeStr=Inherit: Inherit via back propagation  SaturateOnIntegerOverflow=on
  Gain3 : Gain  Gain=IFBK_GAIN  ParamDataTypeStr=fixdt(0,16,16)  OutDataTypeStr=Inherit: Inherit via back propagation  SaturateOnIntegerOverflow=on
  Logical Operator1 : Logic  Inputs=3  AllPortsSameDT=off  OutDataTypeStr=boolean
  Unit Delay2 : UnitDelay  SampleTime=-1
      settings: AttributesFormatString=<initial=%<X0>>\n<tsample=%<SampleTime>>
  Unit Delay3 : UnitDelay  SampleTime=-1
      settings: AttributesFormatString=<initial=%<X0>>\n<tsample=%<SampleTime>>
  Voltage_Limiter : MX_Library/Voltage_Limiter  SystemSampleTime=-1
  Vref_Correction : MX_Library/output_pair_ClosedLoop/Vref_Correction  SystemSampleTime=-1
  control : Stateflow chart
  hc_pair_OpenLoop : MX_Library/hc_pair_OpenLoop  SystemSampleTime=-1  IFBK_MAX=IFBK_MAX  NZ_IFBK=NZ_IFBK  NZ_DUTY=NZ_DUTY  STB_DB_CNT=STB_DB_CNT  OPEN_DB_CNT=OPEN_DB_CNT  OSTG_DB_CNT=OSTG_DB_CNT  STG_DB_CNT=STG_DB_CNT  OC_DB_CNT=OC_DB_CNT
  oc_stg_detection : MX_Library/oc_stg_detection  SystemSampleTime=-1  CD_DEBOUNCE_OPEN_CIRCUIT=OPEN_DB_CNT  CD_DEBOUNCE_SHORT_TO_GROUND=STG_DB_CNT
  hs_cmd : Outport
  ls_cmd : Outport  Port=2
  state_Output : Outport  Port=3  OutDataTypeStr=uint8
  wires:
  Voltage_Limiter/1 -> hc_pair_OpenLoop/1
  Gain3/1 -> Vref_Correction/1
  Vref_Correction/1 -> hc_pair_OpenLoop/6
  ifbk_A2D/1 -> Gain3/1
  Logical Operator1/1 -> hc_pair_OpenLoop/3
  Compare To Constant3/1 -> Logical Operator1/2
  Compare To Constant2/1 -> Logical Operator1/1
  state_VBattery/1 -> Compare To Constant3/1
  FunctionState1/1 -> Compare To Constant2/1
  calc_VBattery/1 -> [calc_VBattery], hc_pair_OpenLoop/5
  afbk_A2D/1 -> Gain2/1
  Gain2/1 -> hc_pair_OpenLoop/4
  hc_pair_OpenLoop/4 -> Unit Delay3/1
  hc_pair_OpenLoop/3 -> Unit Delay2/1
  Unit Delay3/1 -> oc_stg_detection/2  "diag_state"
  Unit Delay2/1 -> oc_stg_detection/1  "oc_state"
  hc_pair_OpenLoop/2 -> ls_cmd/1
  hc_pair_OpenLoop/1 -> hs_cmd/1
  state_Engine/1 -> Compare To Constant5/1
  Compare To Constant5/1 -> Logical Operator1/3
  cmd_Output/1 -> control/1(cmd_Output)
  control/1(state_Output) -> state_Output/1
  control/3(enable_LoSide) -> hc_pair_OpenLoop/2
  enable_STGOffDiag/1 -> control/2(enable_STGOffDiag)
  [ocstg_check] -> control/3(ocstg_check)
  [diag_state] -> control/4(diag_state)
  [ocstg_check] -> hc_pair_OpenLoop/7
  oc_stg_detection/1 -> [diag_state]
  oc_stg_detection/2 -> [ocstg_check]
  ain_PrecRef/1 -> Vref_Correction/2
  control/2(duty_Output) -> Voltage_Limiter/2
  [calc_VBattery] -> Voltage_Limiter/1

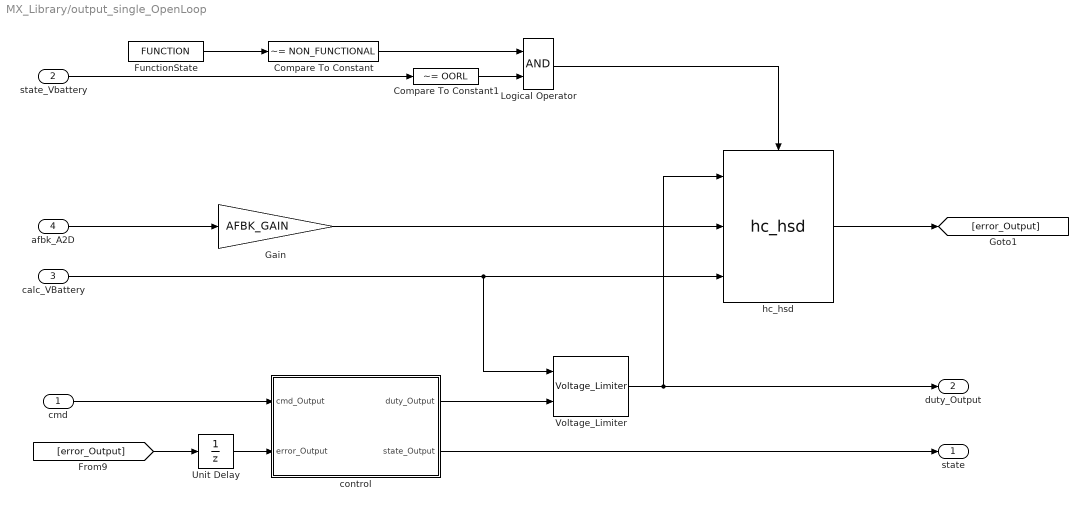
== system MX_Library/output_single_OpenLoop ==
  cmd : Inport
  state_Vbattery : Inport  Port=2
  calc_VBattery : Inport  Port=3
  afbk_A2D : Inport  Port=4  OutDataTypeStr=uint16
  Compare To Constant : simulink/Logic and Bit Operations/Compare To Constant  SystemSampleTime=-1  relop=~=  const=NON_FUNCTIONAL  LogicOutDataTypeMode=boolean  ZeroCross=off
  Compare To Constant1 : simulink/Logic and Bit Operations/Compare To Constant  SystemSampleTime=-1  relop=~=  const=OORL  LogicOutDataTypeMode=boolean  ZeroCross=off
  FunctionState : Constant  Value=FUNCTION  OutDataTypeStr=uint8  SampleTime=-1
  Gain : Gain  Gain=AFBK_GAIN  ParamDataTypeStr=fixdt(0,16,8)  OutDataTypeStr=fixdt(0,16,8)  RndMeth=Zero  SaturateOnIntegerOverflow=on
  Logical Operator : Logic  AllPortsSameDT=off  OutDataTypeStr=boolean
  Unit Delay : UnitDelay  SampleTime=-1
  Voltage_Limiter : MX_Library/Voltage_Limiter  SystemSampleTime=-1
  control : Stateflow chart
  hc_hsd : MX_Library/hc_hsd  SystemSampleTime=-1  STB_DB_CNT=STB_DB_CNT  STG_DB_CNT=STG_DB_CNT  OPEN_DB_CNT=OPEN_DB_CNT
  state : Outport
  duty_Output : Outport  Port=2
  wires:
  Logical Operator/1 -> hc_hsd/Enable
  Compare To Constant1/1 -> Logical Operator/2
  Gain/1 -> hc_hsd/2
  afbk_A2D/1 -> Gain/1
  calc_VBattery/1 -> hc_hsd/3, Voltage_Limiter/1
  Compare To Constant/1 -> Logical Operator/1
  FunctionState/1 -> Compare To Constant/1
  state_Vbattery/1 -> Compare To Constant1/1
  cmd/1 -> control/1(cmd_Output)
  hc_hsd/1 -> [error_Output]
  [error_Output] -> Unit Delay/1
  control/2(state_Output) -> state/1
  Unit Delay/1 -> control/2(error_Output)
  control/1(duty_Output) -> Voltage_Limiter/2
  Voltage_Limiter/1 -> duty_Output/1, hc_hsd/1

== system MX_Library/relay_oc ==
  note: Inputs:
      |     cmd:  desired output (boolean)
      |
      |     fbk:  digital feedback on output pin (boolean)
      |
      | Outputs:
      |     state:   8-bit value representing driver state
      |             (8) -> ok
      |             (2) -> output error on   // cmd==off fbk==on  din==on
      |             (2) -> relay error on    // cmd==off fbk==off din==on
      |             (3) -> output error off  // cmd==on  fbk==off din==off
      |             (3) -> relay error on    // cmd==off fbk==off din==on
      |             (7) -> open circuit      // cmd==off fbk==on  din==off
      |             (28)-> failure           // cmd==on  fbk==off din==on
  cmd : Inport  OutDataTypeStr=boolean
  dfbk : Inport  Port=2  OutDataTypeStr=boolean
  din : Inport  Port=3  OutDataTypeStr=boolean
  Enable : EnablePort
  relay_error_state : Stateflow chart
  state_Output : Outport  OutDataTypeStr=uint8  OutputWhenDisabled=reset  InitialOutput=[8]
  state_Relay : Outport  Port=2  OutDataTypeStr=uint8  OutputWhenDisabled=reset  InitialOutput=[8]
  wires:
  relay_error_state/1(state_Relay) -> state_Relay/1  "state_Relay"
  relay_error_state/2(state_Output) -> state_Output/1  "state_Output"
  cmd/1 -> relay_error_state/1(cmd)  "cmd"
  din/1 -> relay_error_state/3(din)  "din"
  dfbk/1 -> relay_error_state/2(dfbk)  "dfbk"

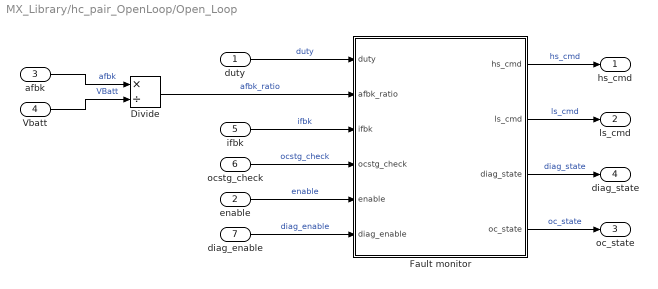
== system MX_Library/hc_pair_OpenLoop/Open_Loop ==
  duty : Inport  OutDataTypeStr=fixdt(0,16,16)
  enable : Inport  Port=2  OutDataTypeStr=boolean
  afbk : Inport  Port=3  OutDataTypeStr=fixdt(0,16,8)
  Vbatt : Inport  Port=4  OutDataTypeStr=fixdt(0,16,8)
  ifbk : Inport  Port=5  OutDataTypeStr=fixdt(0,16,12)
  ocstg_check : Inport  Port=6
  diag_enable : Inport  Port=7  OutDataTypeStr=boolean
  Divide : Product  Inputs=*/  OutDataTypeStr=fixdt(1,16,8)  RndMeth=Simplest  LockScale=on
  Fault monitor : Stateflow chart
  hs_cmd : Outport  OutDataTypeStr=fixdt(0,16,16)
  ls_cmd : Outport  Port=2  OutDataTypeStr=boolean
  oc_state : Outport  Port=3  OutDataTypeStr=uint8  InitialOutput=8
  diag_state : Outport  Port=4  OutDataTypeStr=uint8  InitialOutput=8
  wires:
  diag_enable/1 -> Fault monitor/6(diag_enable)  "diag_enable"
  enable/1 -> Fault monitor/5(enable)  "enable"
  ocstg_check/1 -> Fault monitor/4(ocstg_check)  "ocstg_check"
  duty/1 -> Fault monitor/1(duty)  "duty"
  ifbk/1 -> Fault monitor/3(ifbk)  "ifbk"
  Divide/1 -> Fault monitor/2(afbk_ratio)  "afbk_ratio"
  Fault monitor/4(oc_state) -> oc_state/1  "oc_state"
  Fault monitor/3(diag_state) -> diag_state/1  "diag_state"
  Fault monitor/2(ls_cmd) -> ls_cmd/1  "ls_cmd"
  Fault monitor/1(hs_cmd) -> hs_cmd/1  "hs_cmd"
  Vbatt/1 -> Divide/2  "VBatt"
  afbk/1 -> Divide/1  "afbk"

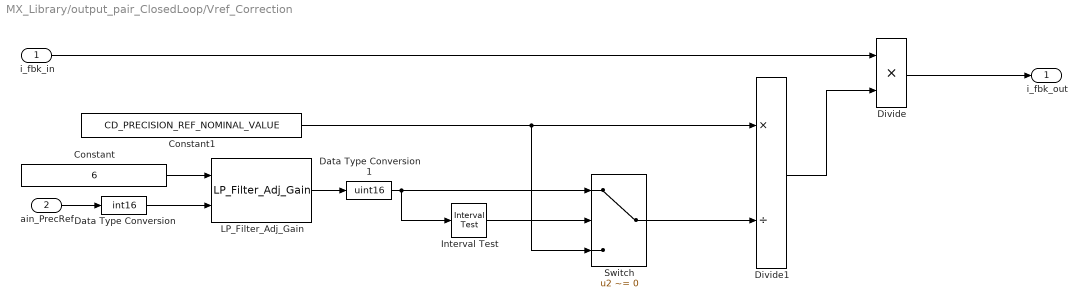
== system MX_Library/output_pair_ClosedLoop/Vref_Correction ==
  i_fbk_in : Inport  OutDataTypeStr=fixdt(0,16,12)
  ain_PrecRef : Inport  Port=2  OutDataTypeStr=uint16
  Constant : Constant  Value=6  OutDataTypeStr=uint8  SampleTime=srate
  Constant1 : Constant  Value=CD_PRECISION_REF_NOMINAL_VALUE  OutDataTypeStr=uint16  SampleTime=srate
  Data Type Conversion : DataTypeConversion  OutDataTypeStr=int16
  Data Type Conversion1 : DataTypeConversion  OutDataTypeStr=uint16
  Divide : Product  Inputs=**  OutDataTypeStr=fixdt(0,16,12)  RndMeth=Simplest
  Divide1 : Product  Inputs=*/  OutDataTypeStr=fixdt(0,16,15)
  Interval Test : simulink/Logic and Bit Operations/Interval Test  SystemSampleTime=-1  IntervalClosedRight=off  uplimit=569  IntervalClosedLeft=off  lowlimit=465  LogicOutDataTypeMode=boolean
  LP_Filter_Adj_Gain : MX_Library/LP_Filter_Adj_Gain  SystemSampleTime=-1
  Switch : Switch  Criteria=u2 ~= 0
  i_fbk_out : Outport
  wires:
  Divide/1 -> i_fbk_out/1
  ain_PrecRef/1 -> Data Type Conversion/1
  Data Type Conversion/1 -> LP_Filter_Adj_Gain/2
  Constant1/1 -> Divide1/1, Switch/3
  i_fbk_in/1 -> Divide/1
  LP_Filter_Adj_Gain/1 -> Data Type Conversion1/1
  Constant/1 -> LP_Filter_Adj_Gain/1
  Interval Test/1 -> Switch/2
  Switch/1 -> Divide1/2
  Data Type Conversion1/1 -> Switch/1, Interval Test/1
  Divide1/1 -> Divide/2

== stateflow chart LP_Filter_Adj_Gain/LP_Filter_Adj_Gain ==
  state INITIAL
    en:Output = Input;
  state LP_FILTER
    du:Output = Output + ((Input - Output)/(1 << Gain));
  (default) -> INITIAL
  INITIAL -> LP_FILTER
  data: Gain input uint8; Input input int16; Output output fixdt(1,32,16)

== stateflow chart LP_Filter_Adj_System/LP_Fitler_Adj_Gain ==
  state INITIAL
    en:Output = Input;
  state LP_FILTER
    du:Output = Output + ((Input - Output)/(1 << Gain));
  (default) -> INITIAL
  INITIAL -> LP_FILTER : [(state_System == 1)]
  data: Gain input uint8; Input input int16; Output output fixdt(1,32,16); state_System input uint8

== stateflow chart relay_oc/relay_error_state ==
  state STATE_OUTPUT [parallel]
    settings: executionOrder=1
    state OUTPUT
      state NORMAL
        state DEBOUNCE
          en: debounceOutput = 0;
          du: debounceOutput++;
        state FAULT
          en: state_Output = NORMAL;
        (default) -> STATE_OUTPUT.OUTPUT.NORMAL.DEBOUNCE
        STATE_OUTPUT.OUTPUT.NORMAL.DEBOUNCE -> STATE_OUTPUT.OUTPUT.NORMAL.FAULT : [(debounceOutput >= NORMAL_DB_CNT)...
            | || (state_Output == NORMAL)]
      state ERROR_ON
        state DEBOUNCE
          en: debounceOutput = 0;
          du: debounceOutput++;
        state FAULT
          en: state_Output = ERROR_ON;
        (default) -> STATE_OUTPUT.OUTPUT.ERROR_ON.DEBOUNCE
        STATE_OUTPUT.OUTPUT.ERROR_ON.DEBOUNCE -> STATE_OUTPUT.OUTPUT.ERROR_ON.FAULT : [(debounceOutput >= ERROR_ON_DB_CNT)...
            | || (state_Output == ERROR_ON)]
      state ERROR_OFF
        state DEBOUNCE
          en: debounceOutput = 0;
          du: debounceOutput++;
        state FAULT
          en: state_Output = ERROR_OFF;
        (default) -> STATE_OUTPUT.OUTPUT.ERROR_OFF.DEBOUNCE
        STATE_OUTPUT.OUTPUT.ERROR_OFF.DEBOUNCE -> STATE_OUTPUT.OUTPUT.ERROR_OFF.FAULT : [(debounceOutput >= ERROR_OFF_DB_CNT)...
            | || (state_Output == ERROR_OFF)]
      state OPEN_CIRCUIT
        state DEBOUNCE
          en: debounceOutput = 0;
          du: debounceOutput++;
        state FAULT
          en: state_Output = OPEN_CIRCUIT;
        (default) -> STATE_OUTPUT.OUTPUT.OPEN_CIRCUIT.DEBOUNCE
        STATE_OUTPUT.OUTPUT.OPEN_CIRCUIT.DEBOUNCE -> STATE_OUTPUT.OUTPUT.OPEN_CIRCUIT.FAULT : [(debounceOutput >= ERROR_OFF_DB_CNT)...
            | || (state_Output == OPEN_CIRCUIT)]
      state FAILURE
        state FAULT
          en: state_Output = FAILURE;
        state DEBOUNCE
          en: debounceOutput = 0;
          du: debounceOutput++;
        (default) -> STATE_OUTPUT.OUTPUT.FAILURE.DEBOUNCE
        STATE_OUTPUT.OUTPUT.FAILURE.DEBOUNCE -> STATE_OUTPUT.OUTPUT.FAILURE.FAULT : [(debounceOutput >= ERROR_OFF_DB_CNT)...
            | || (state_Output == FAILURE)]
      note: The !(din) on Open Circuit and Failure are commented out
          | so full coverage is realized.  That statement will not be executed
          | due to the order of execution as Error on and Failure have the false
          | statement for it covered.
      (default) -> STATE_OUTPUT.OUTPUT.NORMAL : {
          | state_Output = NORMAL;
          | }
      STATE_OUTPUT.OUTPUT.NORMAL -> STATE_OUTPUT.OUTPUT.ERROR_ON [order 1] : [!(cmd)...
          | && (dfbk)...
          | && (din)]
      STATE_OUTPUT.OUTPUT.ERROR_ON -> STATE_OUTPUT.OUTPUT.NORMAL : [((cmd) || !(dfbk) || !(din))...
          | && ((state_Output == NORMAL) || (NORMAL_DB_CNT != UNLIMITED))]
      STATE_OUTPUT.OUTPUT.NORMAL -> FAILURE [order 2] : [(cmd)...
          | && !(dfbk)...
          | && (din)]
      FAILURE -> STATE_OUTPUT.OUTPUT.NORMAL : [(!(cmd) || (dfbk) || !(din))...
          | && ((state_Output == NORMAL) || (NORMAL_DB_CNT != UNLIMITED))]
      STATE_OUTPUT.OUTPUT.NORMAL -> STATE_OUTPUT.OUTPUT.ERROR_OFF [order 3] : [(cmd)...
          | && !(dfbk)
          | /*&& !(din) for coverage*/]
      STATE_OUTPUT.OUTPUT.ERROR_OFF -> STATE_OUTPUT.OUTPUT.NORMAL : [(!(cmd) || (dfbk) || (din))...
          | && ((state_Output == NORMAL) || (NORMAL_DB_CNT != UNLIMITED))]
      STATE_OUTPUT.OUTPUT.NORMAL -> OPEN_CIRCUIT [order 4] : [!(cmd)...
          | && (dfbk)...
          | /*&& !(din) for coverage*/]
      OPEN_CIRCUIT -> STATE_OUTPUT.OUTPUT.NORMAL : [((cmd) || !(dfbk) || (din))...
          | && ((state_Output == NORMAL) || (NORMAL_DB_CNT != UNLIMITED))]
    state RELAY
    note: If the relay state changes we do not want to have an ouptut flag an alarm as well, just one or the
        | other.
    STATE_OUTPUT.OUTPUT -> STATE_OUTPUT.RELAY : [(state_Relay != NORMAL)...
        | && (state_Output == NORMAL)]
    (default) -> STATE_OUTPUT.OUTPUT
    STATE_OUTPUT.RELAY -> STATE_OUTPUT.OUTPUT : [(state_Relay == NORMAL)]
  state STATE_RELAY [parallel]
    settings: executionOrder=2
    state OUTPUT
    note: If the output state changes to be not normal or not failure we do not want to have a relay flag an alarm as well, just one or the
        | other.
    state RELAY
      state NORMAL
        state DEBOUNCE
          en: debounceRelay = 0;
          du: debounceRelay++;
        state FAULT
          en: state_Relay = NORMAL;
        (default) -> STATE_RELAY.RELAY.NORMAL.DEBOUNCE
        STATE_RELAY.RELAY.NORMAL.DEBOUNCE -> STATE_RELAY.RELAY.NORMAL.FAULT : [(debounceRelay >= NORMAL_DB_CNT)...
            | || (state_Relay == NORMAL)]
      state ERROR_OFF
        state FAULT
          en: state_Relay = ERROR_OFF;
        state DEBOUNCE
          en: debounceRelay = 0;
          du: debounceRelay++;
        (default) -> STATE_RELAY.RELAY.ERROR_OFF.DEBOUNCE
        STATE_RELAY.RELAY.ERROR_OFF.DEBOUNCE -> STATE_RELAY.RELAY.ERROR_OFF.FAULT : [(debounceRelay >= ERROR_OFF_DB_CNT)...
            | || (state_Relay == ERROR_OFF)]
      state ERROR_ON
        state DEBOUNCE
          en: debounceRelay = 0;
          du: debounceRelay++;
        state FAULT
          en: state_Relay = ERROR_ON;
        STATE_RELAY.RELAY.ERROR_ON.DEBOUNCE -> STATE_RELAY.RELAY.ERROR_ON.FAULT : [(debounceRelay >= ERROR_ON_DB_CNT)...
            | || (state_Relay == ERROR_ON)]
        (default) -> STATE_RELAY.RELAY.ERROR_ON.DEBOUNCE
      STATE_RELAY.RELAY.ERROR_OFF -> STATE_RELAY.RELAY.NORMAL : [(!(cmd) || (!(dfbk) && (state_Output != FAILURE)) || (din))...
          | && ((state_Relay == NORMAL) || (NORMAL_DB_CNT != UNLIMITED))]
      STATE_RELAY.RELAY.NORMAL -> STATE_RELAY.RELAY.ERROR_OFF [order 2] : [((cmd)...
          | && ((dfbk) || (state_Output == FAILURE))...
          | && !(din))]
      (default) -> STATE_RELAY.RELAY.NORMAL : {
          | state_Relay = NORMAL;
          | }
      STATE_RELAY.RELAY.ERROR_ON -> STATE_RELAY.RELAY.NORMAL : [((cmd) || (dfbk) || !(din))...
          | && ((state_Relay == NORMAL) || (NORMAL_DB_CNT != UNLIMITED))]
      STATE_RELAY.RELAY.NORMAL -> STATE_RELAY.RELAY.ERROR_ON [order 1] : [!(cmd)...
          | && !(dfbk)...
          | && (din)]
    (default) -> STATE_RELAY.RELAY
    STATE_RELAY.RELAY -> STATE_RELAY.OUTPUT : [(state_Output != NORMAL)...
        | && (state_Output != FAILURE)...
        | && (state_Relay == NORMAL)]
    STATE_RELAY.OUTPUT -> STATE_RELAY.RELAY : [(state_Output == NORMAL)...
        | || (state_Output == FAILURE)]
  data: state_Relay output uint8; debounceOutput local uint16; state_Output output uint8; debounceRelay local uint16; ERROR_ON_DB_CNT parameter uint16; NORMAL_DB_CNT parameter uint16; ERROR_OFF_DB_CNT parameter uint16; cmd input boolean; dfbk input boolean; din input boolean; NORMAL parameter uint8; ERROR_ON parameter uint8; ERROR_OFF parameter uint8; OPEN_CIRCUIT parameter uint8; FAILURE parameter uint8; UNLIMITED parameter uint16

== stateflow chart hc_hsd/Fault monitor ==
  settings: sampleTime=0.01
  state OPEN_CIRCUIT
    state DEBOUNCE
      en: db_cnt = 0;
      du: db_cnt++;
    state FAULT
      state = OPEN_CIRCUIT;
    OPEN_CIRCUIT.DEBOUNCE -> OPEN_CIRCUIT.FAULT : [(db_cnt >= OPEN_DB_CNT)]
    (default) -> OPEN_CIRCUIT.DEBOUNCE
  state SHORT_TO_GROUND
    state FAULT
      state = SHORT_TO_GROUND;
    state DEBOUNCE
      en: db_cnt = 0;
      du: db_cnt++;
    SHORT_TO_GROUND.DEBOUNCE -> SHORT_TO_GROUND.FAULT : [(db_cnt >= STG_DB_CNT)]
    (default) -> SHORT_TO_GROUND.DEBOUNCE
  state SHORT_TO_BATTERY
    state DEBOUNCE
      en: db_cnt = 0;
      du: db_cnt++;
    state FAULT
      state = SHORT_TO_BATTERY;
    SHORT_TO_BATTERY.DEBOUNCE -> SHORT_TO_BATTERY.FAULT : [(db_cnt >= STB_DB_CNT)]
    (default) -> SHORT_TO_BATTERY.DEBOUNCE
  state NORMAL
    en: db_cnt = INACTIVE;
    en: state = NORMAL;
  (default) -> NORMAL
  SHORT_TO_GROUND -> NORMAL : [(state == NORMAL)...
      | && ((hs_cmd < 0.98C)...
      |        || (afbk_ratio >= 0.20C))]
  NORMAL -> SHORT_TO_GROUND [order 3] : [(hs_cmd >= 0.98C)...
      | && (afbk_ratio < 0.20C)...
      | && (STG_DB_CNT != UNLIMITED)]
  OPEN_CIRCUIT -> NORMAL : [(state == NORMAL)...
      | && ((hs_cmd != INACTIVE)...
      |        || (afbk_ratio <= 0.25C)...
      |        || (afbk_ratio >= 0.75C))]
  NORMAL -> OPEN_CIRCUIT [order 2] : [(hs_cmd == 0)...
      | && (afbk_ratio > 0.25C)...
      | && (afbk_ratio < 0.75C)...
      | && (OPEN_DB_CNT != UNLIMITED)]
  SHORT_TO_BATTERY -> NORMAL : [(state == NORMAL)...
      | && ((hs_cmd != INACTIVE)...
      |        || (afbk_ratio <= 0.80C))]
  NORMAL -> SHORT_TO_BATTERY [order 1] : [(hs_cmd == INACTIVE)...
      | && (afbk_ratio > 0.80C)...
      | && (STB_DB_CNT != UNLIMITED)]
  data: hs_cmd input fixdt(0,16,16); state output uint8; afbk_ratio input fixdt(1,16,8); STB_DB_CNT parameter uint16; STG_DB_CNT parameter uint16; OPEN_DB_CNT parameter uint16; db_cnt local uint16; NORMAL parameter uint8; INACTIVE parameter uint8; OPEN_CIRCUIT parameter uint8; SHORT_TO_GROUND parameter uint8; SHORT_TO_BATTERY parameter uint8; UNLIMITED parameter uint16
